simulink model "MPC_evasive"  (R2020b)
settings: Solver=FixedStepAuto  StartTime=0  StopTime=12  RelTol=1e-3
values from neighbouring files (symbols this model uses):
  map = [road_edge; blank_map; road_edge]    [InitializeMap_lines.m]
  Ts = 0.05    [InitializeMap_lines.m]    (also in MPC.m)
libraries: Solver_SF x1
settings Model: Creator=ASCL-321  LastModifiedBy=ASCL-321

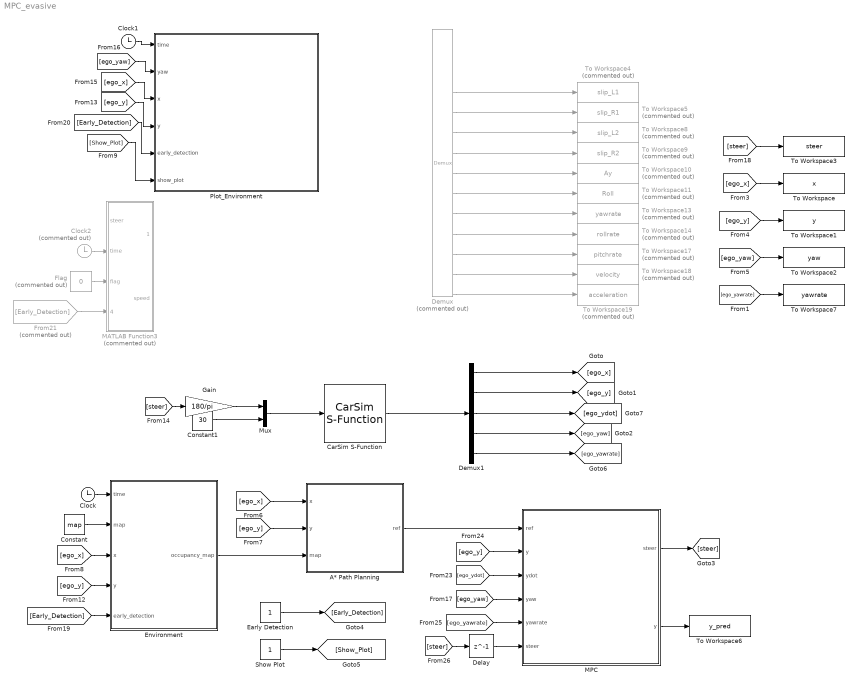
== system MPC_evasive ==
  A* Path Planning : MATLAB Function  TreatAsAtomicUnit=on  SystemSampleTime=Ts
  CarSim S-Function : Solver_SF/CarSim S-Function  Priority=1  SIMFILE=simfile.sim  Run_RTs=off  vs_state_ind=Run  StopMode_ind=Vehicle Model
  Clock : Clock
  Clock1 : Clock
  Clock2 : Clock  Commented=on
  Constant : Constant  Value=map
  Constant1 : Constant  Value=30
  Delay : Delay  DelayLength=1  SampleTime=Ts
  Demux : Demux  Commented=on  Outputs=14
  Demux1 : Demux  Outputs=5
  Early Detection : Constant
  Environment : MATLAB Function  TreatAsAtomicUnit=on  SystemSampleTime=Ts
  Flag : Constant  Commented=on  Value=0
  From21 : From  Commented=on  GotoTag=Early_Detection
  Gain : Gain  Gain=180/pi
  MATLAB Function3 : MATLAB Function  Commented=on  TreatAsAtomicUnit=on
  MPC : MATLAB Function  TreatAsAtomicUnit=on  SystemSampleTime=Ts
  Mux : Mux  Inputs=2
  Plot_Environment : MATLAB Function  TreatAsAtomicUnit=on  SystemSampleTime=0.1
  Show Plot : Constant
  To Workspace : ToWorkspace  VariableName=x  SaveFormat=Timeseries  SampleTime=0.05
  To Workspace1 : ToWorkspace  VariableName=y  SaveFormat=Timeseries  SampleTime=0.05
  To Workspace10 : ToWorkspace  Commented=on  VariableName=Ay  SaveFormat=Timeseries  SampleTime=0.025
  To Workspace11 : ToWorkspace  Commented=on  VariableName=Roll  SaveFormat=Timeseries  SampleTime=0.025
  To Workspace13 : ToWorkspace  Commented=on  VariableName=yawrate  SaveFormat=Timeseries  SampleTime=0.025
  To Workspace14 : ToWorkspace  Commented=on  VariableName=rollrate  SaveFormat=Timeseries  SampleTime=0.025
  To Workspace17 : ToWorkspace  Commented=on  VariableName=pitchrate  SaveFormat=Timeseries  SampleTime=0.025
  To Workspace18 : ToWorkspace  Commented=on  VariableName=velocity  SaveFormat=Timeseries  SampleTime=0.025
  To Workspace19 : ToWorkspace  Commented=on  VariableName=acceleration  SaveFormat=Timeseries  SampleTime=0.025
  To Workspace2 : ToWorkspace  VariableName=yaw  SaveFormat=Timeseries  SampleTime=0.025
  To Workspace3 : ToWorkspace  VariableName=steer  SaveFormat=Timeseries  SampleTime=0.025
  To Workspace4 : ToWorkspace  Commented=on  VariableName=slip_L1  SaveFormat=Timeseries  SampleTime=0.025
  To Workspace5 : ToWorkspace  Commented=on  VariableName=slip_R1  SaveFormat=Timeseries  SampleTime=0.025
  To Workspace6 : ToWorkspace  VariableName=y_pred  SaveFormat=Timeseries  SampleTime=-1
  To Workspace7 : ToWorkspace  VariableName=yawrate  SaveFormat=Timeseries  SampleTime=0.025
  To Workspace8 : ToWorkspace  Commented=on  VariableName=slip_L2  SaveFormat=Timeseries  SampleTime=0.025
  To Workspace9 : ToWorkspace  Commented=on  VariableName=slip_R2  SaveFormat=Timeseries  SampleTime=0.025
  wires:
  CarSim S-Function/1 -> Demux1/1
  [steer] -> Gain/1
  Demux1/1 -> [ego_x]
  Demux1/2 -> [ego_y]
  [ego_x] -> To Workspace/1
  [ego_y] -> To Workspace1/1
  [ego_yaw] -> To Workspace2/1
  [ego_x] -> A* Path Planning/1(x)
  [ego_y] -> A* Path Planning/2(y)
  [ego_yaw] -> MPC/4(yaw)
  MPC/1(steer) -> [steer]
  Environment/1(occupancy_map) -> A* Path Planning/3(map)
  [steer] -> To Workspace3/1
  Constant/1 -> Environment/2(map)
  Clock/1 -> Environment/1(time)
  [ego_x] -> Environment/3(x)
  [ego_y] -> Environment/4(y)
  [Early_Detection] -> Environment/5(early_detection)
  [Early_Detection] -> Plot_Environment/5(early_detection)
  [ego_yaw] -> Plot_Environment/2(yaw)
  Clock1/1 -> Plot_Environment/1(time)
  [ego_x] -> Plot_Environment/3(x)
  [ego_y] -> Plot_Environment/4(y)
  Early Detection/1 -> [Early_Detection]
  A* Path Planning/1(ref) -> MPC/1(ref)
  Demux/6 -> To Workspace8/1
  Demux/4 -> To Workspace4/1
  Demux/5 -> To Workspace5/1
  Demux/7 -> To Workspace9/1
  Demux/8 -> To Workspace10/1
  Demux/9 -> To Workspace11/1
  Show Plot/1 -> [Show_Plot]
  [Show_Plot] -> Plot_Environment/6(show_plot)
  Demux/10 -> To Workspace13/1
  Demux/11 -> To Workspace14/1
  Gain/1 -> Mux/1
  Constant1/1 -> Mux/2
  Demux/12 -> To Workspace17/1
  Demux/13 -> To Workspace18/1
  Demux/14 -> To Workspace19/1
  Demux1/4 -> [ego_yaw]
  Demux1/5 -> [ego_yawrate]
  Demux1/3 -> [ego_ydot]
  [ego_yawrate] -> MPC/5(yawrate)
  [ego_y] -> MPC/2("y ")
  [ego_ydot] -> MPC/3(ydot)
  Mux/1 -> CarSim S-Function/1
  MPC/2(y) -> To Workspace6/1
  [ego_yawrate] -> To Workspace7/1
  [steer] -> Delay/1
  Delay/1 -> MPC/6("steer ")
  Flag/1 -> MATLAB Function3/3(flag)
  From21/1 -> MATLAB Function3/4(detection)
  Clock2/1 -> MATLAB Function3/2(time)

== matlab function MPC_evasive/MATLAB Function3 ==
  data: steer input; time input; steer_output output; flag input; speed output; detection input
function [steer_output, speed]= fcn(steer, time, flag, detection)
if flag
    steer_output=0;
else
    steer_output=steer; 
end

speed = 30;

% if detection == 1
%     if time > 5
%         speed=0;
%     else
%         speed=30;
%     end
% else
%     if time > 5.7
%         speed=0;
%     else
%         speed=30;
%     end
% end

== matlab function MPC_evasive/A* Path Planning ==
  data: x input; ref output; y input; map input
function ref = fcn(x, y, map)
%% Map parameters
res=10;

road_width = 50; % 50m*10
road_length = 100; % 100m*10
number_of_lanes = 3;
lane_width = 3; %3m*10

lane1 = road_width/2 - lane_width;
lane2 = road_width/2;
lane3 = road_width/2 + lane_width;


%% A* Algorithm

ego_length = 3.3;
ego_width = 1.5;

startx = ego_length/2*res;
starty = lane2*res;
goalx = 99*res;
goaly = lane2 *res;

ego_x = round(startx+x*res);
ego_y = round(starty+y*res);

x_path = zeros(166,1);
y_path = zeros(166,1);

x_path_global = zeros(166,1);
y_path_global = zeros(166,1);



for n = 1:166 % 8.3m/s * 1s *2 preview time
    min = 1000000;
    min_i = ego_x;
    min_j = ego_y;
%     ego_x
    for i = ego_x - 4: ego_x + 4
        for j = ego_y - 4: ego_y + 4
            buffer = sqrt((goalx - i)^2 + (goaly - j)^2);
            buffer = buffer + map(j,i)*buffer;
            if (buffer < min)
                min = buffer;
                min_i = i;
                min_j = j;
            end
        end
    end
    ego_x = min_i;
    ego_y = min_j;
    x_path(n) = (ego_x - round(startx+x*res));
    y_path(n) = (ego_y - round(starty+y*res));
    x_path_global(n) = ego_x;
    y_path_global(n) = ego_y;
end

ref_path = [x_path, y_path]';
ref_yaw = zeros(1,length(ref_path)-2);
e=0.00000001;
for i = 1:length(ref_yaw)
    yaw1 = atan((y_path(i+1)-y_path(i))/(x_path(i+1)-x_path(i)+e));
    yaw2 = atan((y_path(i+2)-y_path(i+1))/(x_path(i+2)-x_path(i)+e));
    yaw = (yaw1+yaw2)/2;
    if x_path>=0
        
    elseif y_path>0
        yaw = pi - yaw;
    else
        yaw = -pi + yaw;
    end
    ref_yaw(1,i) = yaw;
end

hold on
plot(x_path_global/res,y_path_global/res, 'k.')
hold off

ref = [ref_path(2,:);
    0 0 ref_yaw];

== matlab function MPC_evasive/Environment ==
  data: time input; occupancy_map output; map input; x input; y input; early_detection input
function occupancy_map = fcn(time, map, x, y, early_detection)
detection = 0;



%% Map parameters
res=10;
TimeStep=0.1;

road_width = 50; % 50m*10
road_length = 100; % 100m*10
number_of_lanes = 3;
lane_width = 3; % 3m*10

lane1 = road_width/2 - lane_width;
lane2 = road_width/2;
lane3 = road_width/2 + lane_width;

%% Target Vehicle
target1x = 50;
target1y = lane3+0.5;
target1_length = 6; % m
target1_width = 2.3; % m

d_safe = 26.6 + target1_length/2; % 8.3m/s * 3.2s (vel * TTC)

for i = target1x*res - d_safe*res : target1x*res + d_safe*res
    for j = round(target1y*res - lane_width*res*(cos(pi*(i-target1x*res)/d_safe/res))) : round(target1y*res + lane_width*res*(cos(pi*(i-target1x*res)/d_safe/res)))
        map(j,i)=1;
    end
end

%% Child

child_length = 0.3; % 30cm
child_width = 0.3; % 30cm
% child_v = 3; % m/s, +y direction in global
child_v = 2;

child_distance_to_target1 = 3; % m

childx = target1x + target1_length/2 + child_distance_to_target1;
childy = target1y + 2;



d_safe = 26.6; % 8.3m/s * 3.2s (vel * TTC)

% Child movement
% if (time>4.7 && time < 6.7)
%    childy = childy - child_v*(time-4.7);
% elseif (time >= 6.7)
%     childy = childy - child_v*2;
% end
% UAV
% if (time>9 && time < 12)
%    childy = childy - child_v*(time-9);
% elseif (time >= 12)
%     childy = childy - child_v*3;
% end

if (time>4 && time < 7)
   childy = childy - child_v*(time-4);
elseif (time >= 7)
    childy = childy - child_v*3;
end

if early_detection == 1 && time>5
    detection = 1;
end

% if (time>10.7)
if (time>5.7)
    detection = 1;
end

if detection == 1
    
    for i = childx*res - d_safe*res : childx*res + d_safe*res
        for j = round(childy*res - lane_width*res*(cos(pi*(i-childx*res)/d_safe/res))) : round(childy*res + lane_width*res*(cos(pi*(i-childx*res)/d_safe/res)))
            map(j,i) = 1 - abs(childy*res - j) / lane_width*res*(cos(pi*(i-childx*res)/d_safe/res)+1)/200;
        end
    end
end


occupancy_map = flipud(map);

== matlab function MPC_evasive/Plot_Environment ==
  data: time input; yaw input; x input; y input; early_detection input; show_plot input
function fcn(time, yaw, x, y, early_detection, show_plot)

if show_plot == 1
    

    figure(1);
    
    detection = 0;

    %% Map parameters
    res=10;
    TimeStep=0.1;

    road_width = 50; % 50m*10
    road_length = 100; % 100m*10
    number_of_lanes = 3;
    lane_width = 3; % 3m*10

    lane3 = road_width/2 - lane_width;
    lane2 = road_width/2;
    lane1 = road_width/2 + lane_width;

    %% Ego Vehicle

    ego_length = 3.3;
    ego_width = 1.5;
    yaw = yaw*pi/180;


    %% Target Vehicle
    target1x = 50;
    target1y = lane3-0.5;
    target1_length = 6; % m
    target1_width = 2.3; % m

    target2x = 41;
    target2y = lane3-0.5;
    target2_length = 6; % m
    target2_width = 2.3; % m
    


    %% Child

    child_length = 0.5; % 50cm
    child_width = 0.5; % 50cm
%     child_v = 3; % m/s, +y direction in global
    child_v = 2;

    child_distance_to_target1 = 3; % m

    childx = target1x + target1_length/2 + child_distance_to_target1;
    childy = target1y-2;



% %     Child movement
%     if (time>4.7 && time < 6.7)
%        childy = childy + child_v*(time-4.7);
%     elseif (time >= 6.7)
%         childy = childy + child_v*2;
%     end

%     if (time>9 && time < 12)
%        childy = childy + child_v*(time-9);
%     elseif (time >= 12)
%         childy = childy + child_v*3;
%     end
    
    if (time>4 && time < 7)
       childy = childy + child_v*(time-4);
    elseif (time >= 7)
        childy = childy + child_v*3;
    end

    childplotx=[childx-child_length/2 childx+child_length/2];
    childploty=[childy-child_width/2 childy+child_width/2];

    if early_detection == 1 && time>5
        detection = 1;
    end
    
%     if (time>10.7)
    if (time>5.7)
        detection = 1;
    end

    %% Draw on map
    road_zero = road_width/2 - number_of_lanes*lane_width/2;
    road_end=[0 road_length];
    line1=[road_zero road_zero];
    line2=[road_zero+lane_width road_zero+lane_width];
    line3=[road_zero+lane_width*2 road_zero+lane_width*2];
    line4=[road_zero+lane_width*3 road_zero+lane_width*3];
    line5=[road_zero+lane_width*4 road_zero+lane_width*4];

    plot(road_end,line1, 'k-','LineWidth',2)
    hold on
    plot(road_end,line2, 'k--','LineWidth',2)
    plot(road_end,line3, 'k-','LineWidth',2)
    plot(road_end,line4, 'k--','LineWidth',2)
    plot(road_end,line5, 'k-','LineWidth',2)

    target1plotx=[target1x-target1_length/2 target1x+target1_length/2];
    target1ploty=[target1y-target1_width/2 target1y+target1_width/2];
    plot([target1plotx(1) target1plotx(2)], [target1ploty(1) target1ploty(1)], 'm')
    plot([target1plotx(1) target1plotx(2)], [target1ploty(2) target1ploty(2)], 'm')
    plot([target1plotx(1) target1plotx(1)], [target1ploty(1) target1ploty(2)], 'm')
    plot([target1plotx(2) target1plotx(2)], [target1ploty(1) target1ploty(2)], 'm')
    text(target1plotx(1)+1,target1ploty(1)-0.5,"Target")
    
    target2plotx=[target2x-target2_length/2 target2x+target2_length/2];
    target2ploty=[target2y-target2_width/2 target2y+target2_width/2];
    plot([target2plotx(1) target2plotx(2)], [target2ploty(1) target2ploty(1)], 'm')
    plot([target2plotx(1) target2plotx(2)], [target2ploty(2) target2ploty(2)], 'm')
    plot([target2plotx(1) target2plotx(1)], [target2ploty(1) target2ploty(2)], 'm')
    plot([target2plotx(2) target2plotx(2)], [target2ploty(1) target2ploty(2)], 'm')
    text(target2plotx(1)+1,target2ploty(1)-0.5,"Target")

    if detection == 1

        plot([childplotx(1) childplotx(2)], [childploty(1) childploty(1)], 'g')
        plot([childplotx(1) childplotx(2)], [childploty(2) childploty(2)], 'g')
        plot([childplotx(1) childplotx(1)], [childploty(1) childploty(2)], 'g')
        plot([childplotx(2) childplotx(2)], [childploty(1) childploty(2)], 'g')
        text(childplotx(1)-1,childploty(1)-0.5,"Child")

    else
        plot([childplotx(1) childplotx(2)], [childploty(1) childploty(1)], 'r')
        plot([childplotx(1) childplotx(2)], [childploty(2) childploty(2)], 'r')
        plot([childplotx(1) childplotx(1)], [childploty(1) childploty(2)], 'r')
        plot([childplotx(2) childplotx(2)], [childploty(1) childploty(2)], 'r')
        text(childplotx(1)-1,childploty(1)-0.5,"Child")
    end

    h=sqrt((ego_length/2)^2+(ego_width/2)^2);
    theta = atan(ego_width/ego_length);
    psi=theta-yaw;
    x=x+1;
    y=y+25;
    x1=x-h*cos(psi);
    y1=y+h*sin(psi);
    x2=x1+ego_length*cos(yaw);
    y2=y1+ego_length*sin(yaw);
    x3=2*x-x2;
    y3=2*y-y2;
    x4=x3+ego_length*cos(yaw);
    y4=y3+ego_length*sin(yaw);

    plot([x1 x2],[y1 y2], 'b')
    plot([x3 x4],[y3 y4], 'b')
    plot([x1 x3],[y1 y3], 'b')
    plot([x2 x4],[y2 y4], 'b')
    text(x3+0.5,y3-0.5,"Ego")

    hold off

    

    xlim([0,100])
    ylim([15,35])
    title('Map')
%     set(gcf, 'Position',  [100, 50, 1700, 340])
    set(gca,'ytick',[])
end
line_map=1;

== matlab function MPC_evasive/MPC ==
  data: ref input; y input; ydot input; steer output; yaw input; yawrate input; steer input; y output
function [steer, y] = fcn(ref, y, ydot, yaw, yawrate, steer)
% MPC parameters
m = 1723.8;
Iz = 4175;
L = 2.7;
lf = 1.24;
lr = L-lf;
Cf = 67248;
Cr = 53248;
Ts = 0.05;

vx = 30*1000/3600;
Tref = 0.3;
alpha = exp(-Ts/Tref);

A = [0 1 0 0;
    0 -2*(Cf+Cr)/m/vx 0 -vx-2*(lf*Cf-lr*Cr)/m/vx;
    0 0 0 1;
    0 -2*(lf*Cf-lr*Cr)/Iz/vx 0 -2*(lf^2*Cf+lr^2*Cr)/Iz/vx];

B = [0;
    2*Cf/m;
    0;
    2*lf*Cf/Iz];
C = [1 0 0 0;
    0 0 1 0];

u_size = 1;
y_size = 2;
x_size = 4;

Ad = eye(x_size) + Ts*A;
Bd = Ts*B;
Cd = C;
Dd = zeros(y_size,u_size);

Q = eye(y_size);
% R = 0.1*eye(u_size);
N1 = 1; % Preferably always 1.
N2 = 5;
Nu = 5;

A = [Ad Bd;
    zeros(u_size,x_size) eye(u_size)];
B = [zeros(x_size,u_size);
    eye(u_size)];
C = [Cd Dd];

F = computeF(A,C,N1,N2);
H = computeH(A,B,C,N1,N2,Nu,y_size,u_size);

Qbar = computeQbar(Q, N1, N2);
% Rbar = computeRbar(R, Nu);
Rbar = 0.5*eye(Nu);
IB = eye(u_size*Nu);
IL = computeIL(u_size, Nu);

P = H'*Qbar*H + Rbar;
P = (P+P')/2;
% AA = [IB; -IB; IL; -IL; H; -H];
AA = [IB; -IB; IL; -IL];

%% States and Inputs

augStates = [y; ydot; yaw; yawrate; steer];

Y = [y; yaw];
% steer
%% MPC with constraints

f = F*augStates;
Ref = computeRef(ref(:, 1:1+N2), Y, y_size, N1, N2, alpha);

b = computeb(f,steer, Ts, Nu, u_size); % Change input constraints inside the function
q = -H'*Qbar*(Ref-f);

Du = quadprog(P,q,AA, b,[],[],[],[],zeros(Nu,1), optimoptions('quadprog','Algorithm','active-set'));


du = Du(u_size,1);
augStates = A*augStates + B*du;
Y = F*augStates + H*Du;

y = Y(1,1);
steer = augStates(5,1);


end

%% Functions

function Ref = computeRef(true_ref, Y, y_size, N1, N2, alpha)
Ref = zeros(y_size * (N2-N1+1), 1);
for i=N1:N2
    Ref(y_size*i-1:y_size*i,1) = true_ref(:,i+1) - alpha^(i+1)*(true_ref(:,1) - Y);
%     Ref(y_size*i-1:y_size*i,1) = true_ref(:,i+1); % No alpha
end
end

function Qbar = computeQbar(Q, N1, N2)
Q_size = size(Q,1);
Qbar = zeros(Q_size*N2);
for i = N1:N2
    for j = N1:N2
        if i == j
            Qbar(Q_size*i-1:Q_size*i,Q_size*j-1:Q_size*j) = Q;
        else
            Qbar(Q_size*i-1:Q_size*i,Q_size*j-1:Q_size*j) = zeros(Q_size);
        end
    end
end

end

% function Rbar = computeRbar(R, Nu)
% R_size = size(R,1);
% Rbar = zeros(R_size*Nu,R_size*Nu);
% for i = 1:Nu
%     for j = 1:Nu
%         if i == j
%             Rbar(i:R_size*i,R_size*j-1:R_size*j) = R;
%         else
%             Rbar(R_size*i-1:R_size*i,R_size*j-1:R_size*j) = zeros(R_size);
%         end
%     end
% end
% end

function IL = computeIL(u_size, Nu)
IL = zeros(Nu);
for i = 1:Nu
    for j = 1:Nu
        if i < j
            IL(i,j) = zeros(u_size);
        else
            IL(i,j) = eye(u_size);
        end
    end
end
end


function b = computeb(f, u, Ts, Nu, u_size)
dumax = 4*pi*Ts;
dumin = -4*pi*Ts;
umax = pi;
umin = -pi;
ymax = [1;
        1];
ymin = [-1;
        -1];

b1 = zeros(Nu,1); b2 = zeros(Nu,1);
b3 = zeros(Nu,1); b4 = zeros(Nu,1);
b5 = zeros(Nu,1); b6 = zeros(Nu,1);

for i = 1:Nu
    b1(i) = dumax;
    b2(i) = -dumin;
    b3(i) = umax - u;
    b4(i) = -(umin - u);
%     b5(u_size*i-1:u_size*i,1) = ymax - f(u_size*i-1:u_size*i,1);
%     b6(u_size*i-1:u_size*i,1) = -(ymin - f(u_size*i-1:u_size*i,1));
end

% b = [b1;b2;b3;b4;b5;b6];
b = [b1;b2;b3;b4];
end

function F = computeF(A,C,N1,N2)
C_row = size(C,1);
C_column = size(C,2);
F = zeros(C_row*N2,C_column);
for i=N1:N2
    F(C_row*i-1:C_row*i,1:C_column) = C*(A^i);
end

end

function H = computeH(A,B,C,N1,N2,Nu, y_size, u_size)
H = zeros(y_size*N2, u_size*Nu);
for j=N1:N2
    for i=1:Nu
        if j<i
            H(y_size*j-1:y_size*j,i:Nu)=zeros(y_size,u_size);
        else
            H(y_size*j-1:y_size*j,i:Nu) = C*A^(j-i)*B;
        end
    end
end
end
